simulink model "oom_model"  (R2025b)
settings: Solver=FixedStepAuto  StartTime=0.0  StopTime=60  FixedStep=0.01  RelTol=1e-3
model workspace (MAT data in the model file):
  S = 16000000
  alloc_on_restart = 396000
  alloc_rate = 50000
  mem_freed = 330000
  mem_per_proc = 330000
  n_procs = 50
  restart_delay = 2

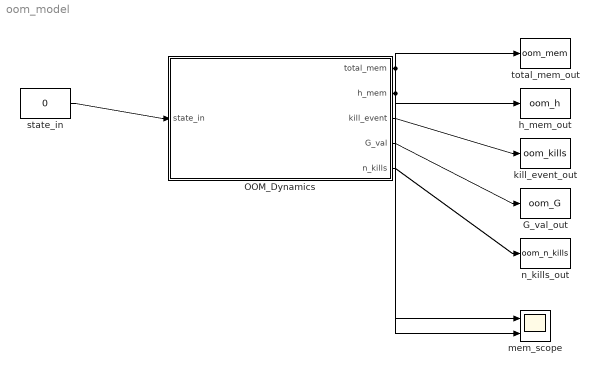
== system oom_model ==
  G_val_out : ToWorkspace  VariableName=oom_G  SaveFormat=Timeseries  SampleTime=-1
  OOM_Dynamics : MATLAB Function  TreatAsAtomicUnit=on
  h_mem_out : ToWorkspace  VariableName=oom_h  SaveFormat=Timeseries  SampleTime=-1
  kill_event_out : ToWorkspace  VariableName=oom_kills  SaveFormat=Timeseries  SampleTime=-1
  mem_scope : Scope  NumInputPorts=2
  n_kills_out : ToWorkspace  VariableName=oom_n_kills  SaveFormat=Timeseries  SampleTime=-1
  state_in : Constant  Value=0
  total_mem_out : ToWorkspace  VariableName=oom_mem  SaveFormat=Timeseries  SampleTime=-1
  wires:
  state_in/1 -> OOM_Dynamics/1(state_in)
  OOM_Dynamics/1(total_mem) -> total_mem_out/1, mem_scope/1
  OOM_Dynamics/2(h_mem) -> h_mem_out/1, mem_scope/2
  OOM_Dynamics/3(kill_event) -> kill_event_out/1
  OOM_Dynamics/4(G_val) -> G_val_out/1
  OOM_Dynamics/5(n_kills) -> n_kills_out/1

== matlab function oom_model/OOM_Dynamics ==
  data: state_in input; total_mem output; h_mem output; kill_event output; G_val output; n_kills output
function [total_mem, h_mem, kill_event, G_val, n_kills] = OOM_Dynamics(state_in)
persistent mem_total kills restart_timer restarting
if isempty(mem_total)
    mem_total = 50 * 330000;  % n_procs * mem_per_proc
    kills = 0;
    restart_timer = -1;
    restarting = false;
end

S = 1.6e+07; mem_freed = 330000; alloc_on_restart = 396000;
restart_delay = 2; alloc_rate = 50000;
dt = 0.01;

% Check OOM condition
kill_event = 0;
if mem_total > S
    mem_total = mem_total - mem_freed;  % kill largest
    kill_event = 1;
    kills = kills + 1;
    restart_timer = restart_delay;  % start restart countdown
    restarting = true;
end

% Restart logic
if restarting
    restart_timer = restart_timer - dt;
    if restart_timer <= 0
        restarting = false;
    end
end

% Post-restart allocation (ramps up)
if ~restarting && restart_timer > -2 && restart_timer <= 0
    mem_total = mem_total + alloc_rate * dt;
    if mem_total >= S  % will trigger OOM again if G >= 1
        restart_timer = -2;  % stop ramping
    end
end

total_mem = mem_total;
h_mem = S - mem_total;
G_val = alloc_on_restart / mem_freed;
n_kills = kills;
